simulink model "sgMdl_IO821_TimeInterrupt"  (R2024b)
settings: Solver=FixedStepAuto  StartTime=0.0  StopTime=inf  RelTol=1e-3  EnableMultiTasking=on
libraries: simulink x2, speedgoatlib_IO821 x2, speedgoatlib_interrupt x1
Description:
  | IO821 - Time Interrupt
settings Model: ModifiedByFormat=Speedgoat  SimulationMode=external  ExtModeTrigDuration=100000  Creator=Speedgoat  LastModifiedBy=Speedgoat
settings SolverCC: ConcurrentTasks=on  AlgebraicLoopSolver=TrustRegion  PositivePriorityOrder=on  InsertRTBMode=Never (minimum delay)
settings DataIOCC: SaveFormat=Array  SaveState=on  SignalLoggingName=logsOut
settings OptimizationCC: BlockReduction=off  BooleanDataType=off  OptimizeBlockIOStorage=off  BufferReuse=off  ReuseModelBlockBuffer=off  GlobalBufferReuse=off  ExpressionFolding=off  LocalBlockOutputs=off  InitFltsAndDblsToZero=on  OptimizeDataStoreBuffers=off  BusAssignmentInplaceUpdate=off
settings DebuggingCC: SaveWithParameterizedLinksMsg=none  UnderspecifiedInitializationDetection=Classic  MergeDetectMultiDrivingBlocksExec=none  CheckExecutionContextPreStartOutputMsg=on  SignalResolutionControl=TryResolveAllWithWarning  TasksWithSamePriorityMsg=none  UnconnectedInputMsg=warning  UnconnectedOutputMsg=warning  UnconnectedLineMsg=warning  SFUnexpectedBacktrackingDiag=warning  SFNoUnconditionalDefaultTransitionDiag=warning  SFExecutionAtInitializationDiag=none  ArithmeticOperatorsInVariantConditions=warning
settings HardwareCC: ProdBitPerLong=64  ProdLongLongMode=on  ProdHWDeviceType=Intel->x86-64 (Linux 64)
settings ModelReferenceCC: EnableRefExpFcnMdlSchedulingChecks=on  PropagateSignalLabelsOutOfModel=off
settings SFSimCC: SimUseLocalCustomCode=off  SimTargetLang=C++
settings RTWCC: Description=Speedgoat Real-Time Target Machine  SystemTargetFile=speedgoat.tlc  TemplateMakefile=slrealtime_default_tmf  PostCodeGenCommand=sg.model.build.makeCfg(bdroot, buildInfo);  RTWUseLocalCustomCode=off  Toolchain=Simulink Real-Time Toolchain  BuildConfiguration=Faster Runs  TargetLang=C++  GPUComputeCapability=3.5  DLArmComputeVersion=19.05
settings CodeAppCC: StateflowObjectComments=on
settings SimulinkRealTimeTargetCC: SubcomponentCodeInterfacePackaging=Reusable function  MATLABClassNameForMDSCustomization=Simulink.SoftwareTarget.GRTCustomization  InstructionSetFMA=off  LogToMDFFile=off  SLRTFileLogMaxRuns=10  UseGCCFastMath=on
settings ConfigComp: CovMetricSettings=dw  CovSaveCumulativeToWorkspaceVar=on  CovSaveSingleToWorkspaceVar=on  CovExternalEMLEnable=off  CovSFcnEnable=off  CovBoundaryAbsTol=1.0e-5

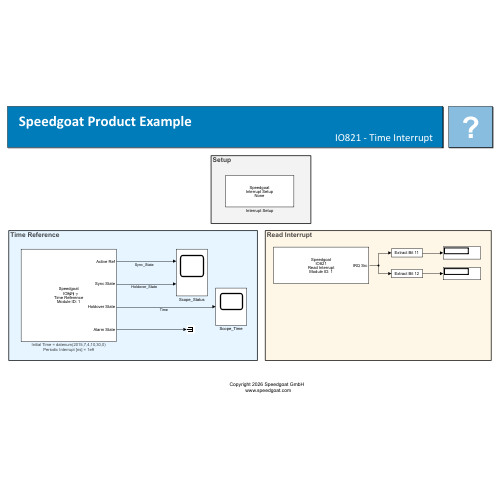
[thumbnail: Simulink's stored preview of the top-level diagram]
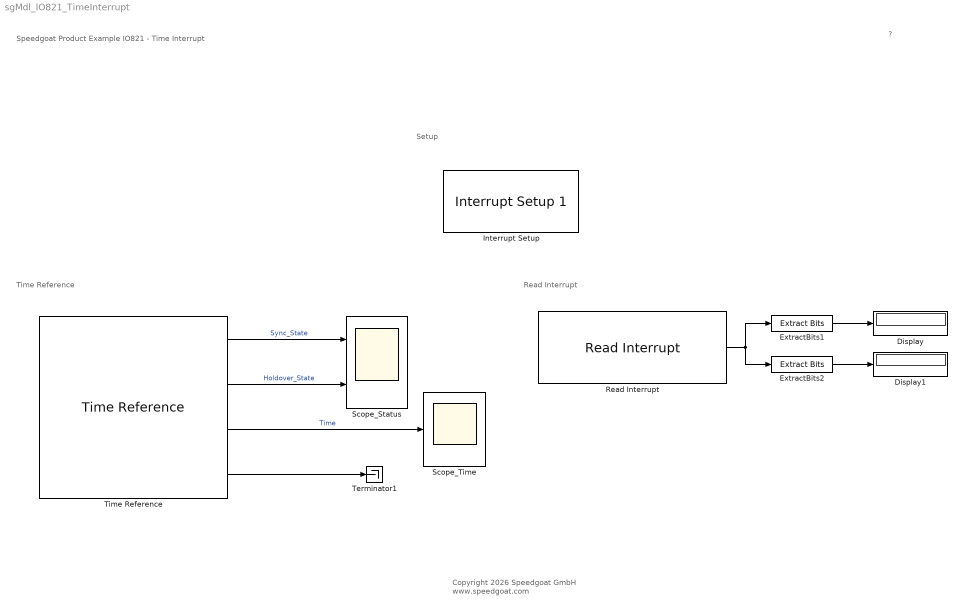
== system sgMdl_IO821_TimeInterrupt ==
  note: Read Interrupt
  note: Setup
  note: Time Reference
  note: Speedgoat Product Example
      | IO821 - Time Interrupt
  note: ?
  note: Copyright 2026 Speedgoat GmbH
      |  www.speedgoat.com
  Display : Display
  Display1 : Display
  ExtractBits1 : simulink/Logic and Bit Operations/Extract Bits  bitsToExtract=Range of bits  numBits=8  bitIdxRange=[11]  outScalingMode=Treat bit field as an integer
  ExtractBits2 : simulink/Logic and Bit Operations/Extract Bits  bitsToExtract=Range of bits  numBits=8  bitIdxRange=[12]  outScalingMode=Treat bit field as an integer
  Interrupt Setup : speedgoatlib_interrupt/Interrupt Setup 1  parModuleTrigger=on  parPollingMode=off  parPriorityConf=High  parPriority=254  confStartFcn=IO821_start_public  confStopFcn=IO821_stop_public  confIsrFcn=IO821_isr_public  confMapFcn=IO821_map_public  confHookFile=io821_int_hooks.c  confIrqNr=-1  confIsPolling=off  confModID=16776961  confSelectedInt=Speedgoat IO821 interrupt  confSelectedId=1  confSelectedChannel=[]  confData=[]  confForcePollingMode=off
  Read Interrupt : speedgoatlib_IO821/Read Interrupt  parModuleId=1  parSampleTime=-1
      settings: SourceProductName=Simulink Real-Time: Speedgoat I/O Blockset
  Scope_Status : Scope  NumInputPorts=2
  Scope_Time : Scope
  Terminator1 : Terminator
  "Time Reference " : speedgoatlib_IO821/Time Reference   parPciSlot=-1  parModuleId=1  parPeriodicIntEnable=on  parNanoPeriod=1e9  parIntDutyCycle=50  parPeriodicIntAlign=off  parLeadTime1=0  parShowSyncState=on  parShowHoldoverState=on  parShowAlarmState=off  parShowTime=on  parOutputFormat=MATLAB datenum/subsec  parTimeOffset=+/-0  parInitialTime=datenum(2015,7,4,10,30,0)  parInitialTime_adapted=datenum(2015,7,4,10,30,0)  par0EdgeDetection=off  par1EdgeDetection=off  parEdgeDetectionFormat=[YYYY,MM,DD,hh,mm,ss]/microseconds of year  par0SignalEdge=Rising Edge  par1SignalEdge=Rising Edge  parHwTrig1Enable=off  parHwTrig1Edge=Rising Edge  parHwTrig1LeadTime=0  parHwTrig2Enable=off  parHwTrig2Edge=Rising Edge  parHwTrig2LeadTime=0  parIRIGenable=on  parLeadTime2=0  parIRIGexpression=BCD TOY, Control Functions, Binary Seconds (SBS)  parCFconfig=RCC 200 - 04  parRefEnable_1=on  parRefPrio_1=1  parRefTime_1=Initial Module Time  parRef1PPS_1=Self Referenced  parRefEnable_2=off  parRefPrio_2=2  parRefTime_2=IRIG DCLS  parRef1PPS_2=IRIG DCLS  parRefEnable_3=off  parRefPrio_3=3  parRefTime_3=IRIG AM  parRef1PPS_3=IRIG AM  parRefEnable_4=off  parRefPrio_4=4  parRefTime_4=IRIG AM  parRef1PPS_4=External 1PPS  parRefEnable_5=off  parRefPrio_5=5  parRefTime_5=Initial Module Time  parRef1PPS_5=External 1PPS  parRefEnable_6=off  parRefPrio_6=6  parRefTime_6=Initial Module Time  parRef1PPS_6=Self Referenced  parShowActiveRef=off
      settings: SourceProductName=Simulink Real-Time: Speedgoat I/O Blockset
      settings: AttributesFormatString=|
      | Initial Time = %<parInitialTime>
      | Periodic Interrupt [ns] = %<parNanoPeriod>
  wires:
  "Time Reference "/2 -> Scope_Status/2  "Holdover_State"
  "Time Reference "/1 -> Scope_Status/1  "Sync_State"
  Read Interrupt/1 -> ExtractBits1/1, ExtractBits2/1
  "Time Reference "/3 -> Scope_Time/1  "Time"
  "Time Reference "/4 -> Terminator1/1
  ExtractBits1/1 -> Display/1
  ExtractBits2/1 -> Display1/1
